simulink model "mavsim_fuzzy"  (R2018b)
settings: Solver=ode15s  StartTime=0  StopTime=50  FixedStep=P.Ts  MaxStep=0.01  RelTol=1e-3  EnableMultiTasking=on
InitFcn:
  | aerosonde
  | param_chap7
values from neighbouring files (symbols this model uses):
  F = [         1, 2, 3, 1;         1, 3, 4, 1;         1, 2, 5, 1;         1, 5, 4, 1;         2, 3, 6, 2;         3, 4, 6, 3;         2, 5, 6, 2;         4, 5, 6, 4;         6, 15, 16, 6;         7, 8, 9, 10;         11, 12, 13, 14;         ]    [drawVehicle.m]    (also in draw_runway.m)
  q = uu(11)    [drawVehicle.m]    (also in forceee.m; plotmavstatevariables.m = 180/pi*uu(11); plotresults.m = 180/pi*uu(11))
  r = uu(12)    [drawVehicle.m]    (also in forceee.m; plotmavstatevariables.m = 180/pi*uu(12); plotresults.m = 180/pi*uu(12))
undefined symbols (not defined in the file or in its folder): altitude_state_machine, drawVehicle, forceee, forces_moments, gps, Light, MIL, P, plotmavstatevariables, plotresults, sensors, true_states
libraries: fuzblock x10, simulink_extras x9, aerolibwind2 x4, sharedtransform x2, simulink x2, aerolibobsolete x1
(part 2 of 2)

== system mavsim_fuzzy/Autopilot/Pitch Loop PD fuzzy/fuzzy elevator2 ==
  Bus Selector2 : BusSelector  OutputSignals=h_c,h,Va,Va_c
  Constant : Constant  Value=0
  Degrees to Radians : simulink_extras/Transformations/Degrees to Radians
  Fuzzy Logic Controller with Ruleviewer : fuzblock/Fuzzy Logic  Controller  with Ruleviewer  fismatrix=P.fuzzy_e2  Ts=2
  Gain : Gain  Gain=-1
  Manual Switch : ManualSwitch
  Mux4 : Mux  Inputs=2
  Sum1 : Sum  Inputs=|-+
  Sum2 : Sum  Inputs=|+-
  delta_e : Outport
  wires:
  [N] -> Bus Selector2/1
  Mux4/1 -> Fuzzy Logic Controller with Ruleviewer/1
  Sum1/1 -> Mux4/1
  Fuzzy Logic Controller with Ruleviewer/1 -> Degrees to Radians/1
  Degrees to Radians/1 -> Gain/1
  Gain/1 -> delta_e/1
  Bus Selector2/1 -> Sum1/1  "<h_c>"
  Bus Selector2/2 -> Sum1/2  "<h>"
  Sum2/1 -> Mux4/2
  Bus Selector2/4 -> Sum2/2  "<Va_c>"
  Constant/1 -> Manual Switch/2
  Bus Selector2/3 -> Manual Switch/1  "<Va>"
  Manual Switch/1 -> Sum2/1

== system mavsim_fuzzy/Autopilot/Pitch Loop PD fuzzy1/fuzzy elevator ==
  Bus Selector2 : BusSelector  OutputSignals=h_c,h,Va,Va_c
  Constant : Constant  Value=0
  Degrees to Radians : simulink_extras/Transformations/Degrees to Radians
  Fuzzy Logic Controller with Ruleviewer : fuzblock/Fuzzy Logic  Controller  with Ruleviewer  fismatrix=P.fuzzy_e  Ts=2
  Gain : Gain  Gain=-1
  Manual Switch : ManualSwitch
  Mux4 : Mux  Inputs=2
  Sum1 : Sum  Inputs=|-+
  Sum2 : Sum  Inputs=|-+
  delta_e : Outport
  wires:
  [N] -> Bus Selector2/1
  Mux4/1 -> Fuzzy Logic Controller with Ruleviewer/1
  Sum1/1 -> Mux4/1
  Fuzzy Logic Controller with Ruleviewer/1 -> Degrees to Radians/1
  Degrees to Radians/1 -> Gain/1
  Gain/1 -> delta_e/1
  Bus Selector2/1 -> Sum1/1  "<h_c>"
  Bus Selector2/2 -> Sum1/2  "<h>"
  Sum2/1 -> Mux4/2
  Bus Selector2/4 -> Sum2/2  "<Va_c>"
  Constant/1 -> Manual Switch/2
  Bus Selector2/3 -> Manual Switch/1  "<Va>"
  Manual Switch/1 -> Sum2/1

== system mavsim_fuzzy/Autopilot/Pitch Loop PD fuzzy1/fuzzy elevator2 ==
  Bus Selector2 : BusSelector  OutputSignals=h_c,h,Va,Va_c
  Constant : Constant  Value=0
  Degrees to Radians : simulink_extras/Transformations/Degrees to Radians
  Fuzzy Logic Controller with Ruleviewer : fuzblock/Fuzzy Logic  Controller  with Ruleviewer  fismatrix=P.fuzzy_e2  Ts=2
  Gain : Gain  Gain=-1
  Manual Switch : ManualSwitch
  Mux4 : Mux  Inputs=2
  Sum1 : Sum  Inputs=|-+
  Sum2 : Sum  Inputs=|+-
  delta_e : Outport
  wires:
  [N] -> Bus Selector2/1
  Mux4/1 -> Fuzzy Logic Controller with Ruleviewer/1
  Sum1/1 -> Mux4/1
  Fuzzy Logic Controller with Ruleviewer/1 -> Degrees to Radians/1
  Degrees to Radians/1 -> Gain/1
  Gain/1 -> delta_e/1
  Bus Selector2/1 -> Sum1/1  "<h_c>"
  Bus Selector2/2 -> Sum1/2  "<h>"
  Sum2/1 -> Mux4/2
  Bus Selector2/4 -> Sum2/2  "<Va_c>"
  Constant/1 -> Manual Switch/2
  Bus Selector2/3 -> Manual Switch/1  "<Va>"
  Manual Switch/1 -> Sum2/1

== system mavsim_fuzzy/Autopilot/Throttle Control/Airspeed Hold Using Throttle PI Control ==
  Altitude State Check : Subsystem
  Bus Selector3 : BusSelector  OutputSignals=Va_c,Va
  Sum : Sum  Inputs=|++
  Sum4 : Sum  Inputs=|+-
  course_ki : TransferFcn  Numerator=[P.airspeed_throttle_ki]  Denominator=[1 0]
  course_kp : TransferFcn  Numerator=[P.airspeed_throttle_kp]  Denominator=[0 1]
  delta_t : Outport
  wires:
  Bus Selector3/2 -> Sum4/2  "<Va>"
  [N] -> Bus Selector3/1
  Bus Selector3/1 -> Sum4/1  "<Va_c>"
  Sum4/1 -> Altitude State Check/1(err_in)
  Altitude State Check/1(err_out) -> course_kp/1, course_ki/1  "e_beta"
  Sum/1 -> delta_t/1
  course_kp/1 -> Sum/2
  course_ki/1 -> Sum/1

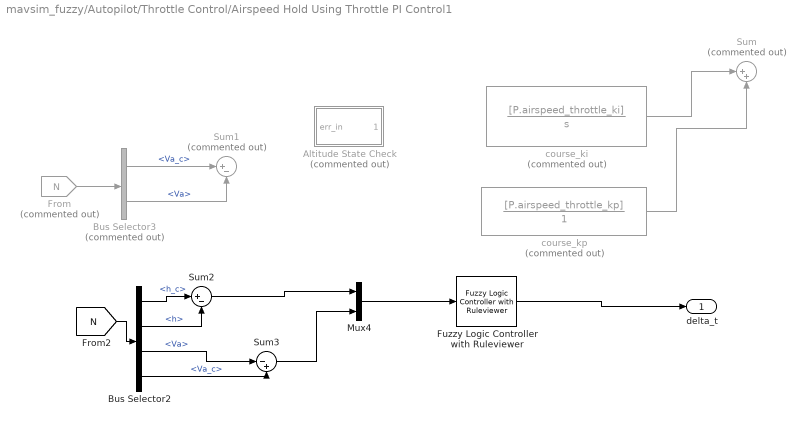
== system mavsim_fuzzy/Autopilot/Throttle Control/Airspeed Hold Using Throttle PI Control1 ==
  Altitude State Check : Subsystem  Commented=on
  Bus Selector2 : BusSelector  OutputSignals=h_c,h,Va,Va_c
  Bus Selector3 : BusSelector  Commented=on  OutputSignals=Va_c,Va
  From : From  Commented=on  GotoTag=N  TagVisibility=global
  Fuzzy Logic Controller with Ruleviewer : fuzblock/Fuzzy Logic  Controller  with Ruleviewer  fismatrix=P.fuzzy_throttle  Ts=2
  Mux4 : Mux  Inputs=2
  Sum : Sum  Commented=on  Inputs=|++
  Sum1 : Sum  Commented=on  Inputs=|+-
  Sum2 : Sum  Inputs=|+-
  Sum3 : Sum  Inputs=|-+
  course_ki : TransferFcn  Commented=on  Numerator=[P.airspeed_throttle_ki]  Denominator=[1 0]
  course_kp : TransferFcn  Commented=on  Numerator=[P.airspeed_throttle_kp]  Denominator=[0 1]
  delta_t : Outport
  wires:
  From/1 -> Bus Selector3/1
  course_kp/1 -> Sum/2
  course_ki/1 -> Sum/1
  Bus Selector3/1 -> Sum1/1  "<Va_c>"
  Bus Selector3/2 -> Sum1/2  "<Va>"
  Mux4/1 -> Fuzzy Logic Controller with Ruleviewer/1
  Bus Selector2/3 -> Sum3/1  "<Va>"
  Sum2/1 -> Mux4/1
  Bus Selector2/2 -> Sum2/2  "<h>"
  Bus Selector2/4 -> Sum3/2  "<Va_c>"
  Bus Selector2/1 -> Sum2/1  "<h_c>"
  [N] -> Bus Selector2/1
  Sum3/1 -> Mux4/2
  Fuzzy Logic Controller with Ruleviewer/1 -> delta_t/1

== system mavsim_fuzzy/Autopilot/Pitch Command Control/Airspeed Hold Using Pitch Loop PI Control/Altitude State Check ==
  err_in : Inport
  Climb Zone : Constant  Value=2
  Product : Product
  Relational Operator : RelationalOperator  Operator===  OutDataTypeStr=boolean  RndMeth=Simplest
  err_out : Outport
  wires:
  err_in/1 -> Product/2
  Relational Operator/1 -> Product/1
  Product/1 -> err_out/1
  [alt_state] -> Relational Operator/1
  Climb Zone/1 -> Relational Operator/2

== system mavsim_fuzzy/Autopilot/Pitch Command Control/Airspeed Hold Using Pitch Loop PI Control /Altitude State Check ==
  err_in : Inport
  Descend Zone : Constant  Value=4
  Product : Product
  Relational Operator : RelationalOperator  Operator===  OutDataTypeStr=boolean  RndMeth=Simplest
  err_out : Outport
  wires:
  err_in/1 -> Product/2
  Relational Operator/1 -> Product/1
  Product/1 -> err_out/1
  [alt_state] -> Relational Operator/1
  Descend Zone/1 -> Relational Operator/2

== system mavsim_fuzzy/Autopilot/Pitch Command Control/Altitude Hold Using Pitch Loop PI Control/Altitude State Check ==
  err_in : Inport
  Alt Hold Zone : Constant  Value=3
  Product : Product
  Relational Operator : RelationalOperator  Operator===  OutDataTypeStr=boolean  RndMeth=Simplest
  err_out : Outport
  wires:
  err_in/1 -> Product/2
  Relational Operator/1 -> Product/1
  Product/1 -> err_out/1
  [alt_state] -> Relational Operator/1
  Alt Hold Zone/1 -> Relational Operator/2

== system mavsim_fuzzy/Autopilot/Pitch Command Control1/Airspeed Hold Using Pitch Loop PI Control/Altitude State Check ==
  err_in : Inport
  Climb Zone : Constant  Value=2
  Product : Product
  Relational Operator : RelationalOperator  Operator===  OutDataTypeStr=boolean  RndMeth=Simplest
  err_out : Outport
  wires:
  err_in/1 -> Product/2
  Relational Operator/1 -> Product/1
  Product/1 -> err_out/1
  [alt_state] -> Relational Operator/1
  Climb Zone/1 -> Relational Operator/2

== system mavsim_fuzzy/Autopilot/Pitch Command Control1/Airspeed Hold Using Pitch Loop PI Control /Altitude State Check ==
  err_in : Inport
  Descend Zone : Constant  Value=4
  Product : Product
  Relational Operator : RelationalOperator  Operator===  OutDataTypeStr=boolean  RndMeth=Simplest
  err_out : Outport
  wires:
  err_in/1 -> Product/2
  Relational Operator/1 -> Product/1
  Product/1 -> err_out/1
  [alt_state] -> Relational Operator/1
  Descend Zone/1 -> Relational Operator/2

== system mavsim_fuzzy/Autopilot/Pitch Command Control1/Altitude Hold Using Pitch Loop PI Control/Altitude State Check ==
  err_in : Inport
  Alt Hold Zone : Constant  Value=3
  Product : Product
  Relational Operator : RelationalOperator  Operator===  OutDataTypeStr=boolean  RndMeth=Simplest
  err_out : Outport
  wires:
  err_in/1 -> Product/2
  Relational Operator/1 -> Product/1
  Product/1 -> err_out/1
  [alt_state] -> Relational Operator/1
  Alt Hold Zone/1 -> Relational Operator/2

== system mavsim_fuzzy/Autopilot/Pitch Command Control2/Airspeed Hold Using Pitch Loop PI Control/Altitude State Check ==
  err_in : Inport
  Climb Zone : Constant  Value=2
  Product : Product
  Relational Operator : RelationalOperator  Operator===  OutDataTypeStr=boolean  RndMeth=Simplest
  err_out : Outport
  wires:
  err_in/1 -> Product/2
  Relational Operator/1 -> Product/1
  Product/1 -> err_out/1
  [alt_state] -> Relational Operator/1
  Climb Zone/1 -> Relational Operator/2

== system mavsim_fuzzy/Autopilot/Pitch Command Control2/Airspeed Hold Using Pitch Loop PI Control /Altitude State Check ==
  err_in : Inport
  Descend Zone : Constant  Value=4
  Product : Product
  Relational Operator : RelationalOperator  Operator===  OutDataTypeStr=boolean  RndMeth=Simplest
  err_out : Outport
  wires:
  err_in/1 -> Product/2
  Relational Operator/1 -> Product/1
  Product/1 -> err_out/1
  [alt_state] -> Relational Operator/1
  Descend Zone/1 -> Relational Operator/2

== system mavsim_fuzzy/Autopilot/Pitch Command Control2/Altitude Hold Using Pitch Loop PI Control/Altitude State Check ==
  err_in : Inport
  Alt Hold Zone : Constant  Value=3
  Product : Product
  Relational Operator : RelationalOperator  Operator===  OutDataTypeStr=boolean  RndMeth=Simplest
  err_out : Outport
  wires:
  err_in/1 -> Product/2
  Relational Operator/1 -> Product/1
  Product/1 -> err_out/1
  [alt_state] -> Relational Operator/1
  Alt Hold Zone/1 -> Relational Operator/2

== system mavsim_fuzzy/Autopilot/Pitch Command Control3/Airspeed Hold Using Pitch Loop PI Control/Altitude State Check ==
  err_in : Inport
  Climb Zone : Constant  Value=2
  Product : Product
  Relational Operator : RelationalOperator  Operator===  OutDataTypeStr=boolean  RndMeth=Simplest
  err_out : Outport
  wires:
  err_in/1 -> Product/2
  Relational Operator/1 -> Product/1
  Product/1 -> err_out/1
  [alt_state] -> Relational Operator/1
  Climb Zone/1 -> Relational Operator/2

== system mavsim_fuzzy/Autopilot/Pitch Command Control3/Airspeed Hold Using Pitch Loop PI Control /Altitude State Check ==
  err_in : Inport
  Descend Zone : Constant  Value=4
  Product : Product
  Relational Operator : RelationalOperator  Operator===  OutDataTypeStr=boolean  RndMeth=Simplest
  err_out : Outport
  wires:
  err_in/1 -> Product/2
  Relational Operator/1 -> Product/1
  Product/1 -> err_out/1
  [alt_state] -> Relational Operator/1
  Descend Zone/1 -> Relational Operator/2

== system mavsim_fuzzy/Autopilot/Pitch Command Control3/Altitude Hold Using Pitch Loop PI Control/Altitude State Check ==
  err_in : Inport
  Alt Hold Zone : Constant  Value=3
  Product : Product
  Relational Operator : RelationalOperator  Operator===  OutDataTypeStr=boolean  RndMeth=Simplest
  err_out : Outport
  wires:
  err_in/1 -> Product/2
  Relational Operator/1 -> Product/1
  Product/1 -> err_out/1
  [alt_state] -> Relational Operator/1
  Alt Hold Zone/1 -> Relational Operator/2

== system mavsim_fuzzy/Autopilot/Throttle Control/Airspeed Hold Using Throttle PI Control/Altitude State Check ==
  err_in : Inport
  Alt Hold Zone : Constant  Value=3
  Product : Product
  Relational Operator : RelationalOperator  Operator===  OutDataTypeStr=boolean  RndMeth=Simplest
  err_out : Outport
  wires:
  err_in/1 -> Product/2
  Relational Operator/1 -> Product/1
  Product/1 -> err_out/1
  [alt_state] -> Relational Operator/1
  Alt Hold Zone/1 -> Relational Operator/2

== system mavsim_fuzzy/Autopilot/Throttle Control/Airspeed Hold Using Throttle PI Control1/Altitude State Check ==
  err_in : Inport
  Alt Hold Zone : Constant  Value=3
  Product : Product
  Relational Operator : RelationalOperator  Operator===  OutDataTypeStr=boolean  RndMeth=Simplest
  err_out : Outport
  wires:
  err_in/1 -> Product/2
  Relational Operator/1 -> Product/1
  Product/1 -> err_out/1
  [alt_state] -> Relational Operator/1
  Alt Hold Zone/1 -> Relational Operator/2
